simulink model "Problem2"  (R2020b)
settings: Solver=VariableStepAuto  StartTime=start_time  StopTime=end_time  RelTol=1e-3
values from neighbouring files (symbols this model uses):
  b = 2500    [Suspension_initial_values.m]
  k1 = 21000    [Suspension_initial_values.m]
  k2 = 320    [Suspension_initial_values.m]
  M1 = 1200    [Suspension_initial_values.m]
  M2 = 13    [Suspension_initial_values.m]
settings Model: Creator=HP  LastModifiedBy=HP

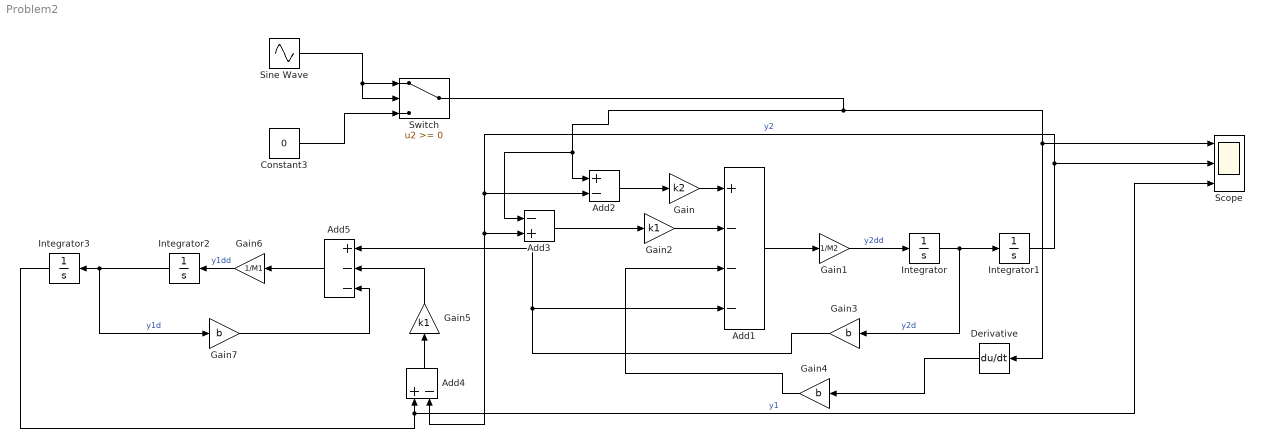
== system Problem2 ==
  Add1 : Sum  Inputs=+---
  Add2 : Sum  Inputs=+-
  Add3 : Sum  Inputs=-+
  Add4 : Sum  Inputs=+-
  Add5 : Sum  Inputs=+--
  Constant3 : Constant  Value=0
  Derivative : Derivative
  Gain : Gain  Gain=k2
  Gain1 : Gain  Gain=1/M2
  Gain2 : Gain  Gain=k1
  Gain3 : Gain  Gain=b
  Gain4 : Gain  Gain=b
  Gain5 : Gain  Gain=k1
  Gain6 : Gain  Gain=1/M1
  Gain7 : Gain  Gain=b
  Integrator{,1..3} (4 alike) : Integrator
  Scope : Scope  NumInputPorts=3
  Sine Wave : Sin  Frequency=0.1  SampleTime=0
  Switch : Switch
  wires:
  Gain/1 -> Add1/1
  Add1/1 -> Gain1/1
  Gain1/1 -> Integrator/1  "y2dd"
  Integrator/1 -> Integrator1/1, Gain3/1  "y2d"
  Integrator1/1 -> Scope/2, Add4/2, Add3/2, Add2/2  "y2"
  Add2/1 -> Gain/1
  Add3/1 -> Gain2/1
  Gain2/1 -> Add1/2
  Derivative/1 -> Gain4/1
  Gain3/1 -> Add1/4, Add5/1
  Gain4/1 -> Add1/3
  Add4/1 -> Gain5/1
  Add5/1 -> Gain6/1
  Gain6/1 -> Integrator2/1  "y1dd"
  Integrator2/1 -> Gain7/1, Integrator3/1  "y1d"
  Integrator3/1 -> Scope/3, Add4/1  "y1"
  Gain7/1 -> Add5/3
  Gain5/1 -> Add5/2
  Switch/1 -> Add3/1, Add2/1, Scope/1, Derivative/1
  Constant3/1 -> Switch/3
  Sine Wave/1 -> Switch/2, Switch/1
